simulink model "Simple_RC_Circuit"  (R2024b)
settings: Solver=VariableStepAuto  StartTime=0.0  StopTime=10.0  RelTol=1e-3
values from neighbouring files (symbols this model uses):
  C = 1e-6    (= 1e-06)    [Simple_RC_Circuit_scripit.m]
  R = i    [Simple_RC_Circuit_scripit.m]
settings Model: Creator=Ahmad  LastModifiedBy=Ahmad

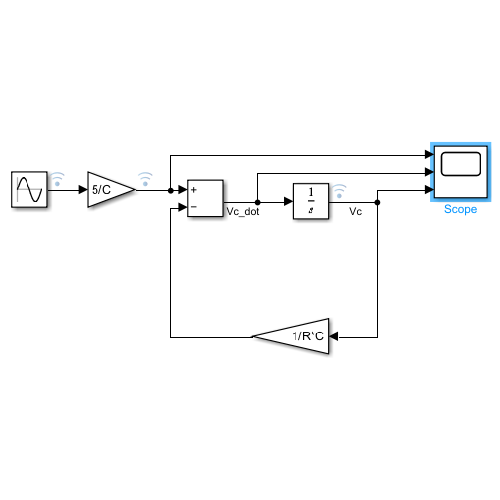
[thumbnail: Simulink's stored preview of the top-level diagram]
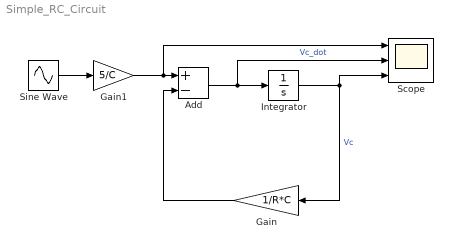
== system Simple_RC_Circuit ==
  Add : Sum  Inputs=+-
  Gain : Gain  Gain=1/R*C
  Gain1 : Gain  Gain=5/C
  Integrator : Integrator
  Scope : Scope  NumInputPorts=3
  Sine Wave : Sin  SampleTime=0
  wires:
  Integrator/1 -> Gain/1, Scope/3  "Vc"
  Gain/1 -> Add/2
  Gain1/1 -> Scope/1, Add/1
  Sine Wave/1 -> Gain1/1
  Add/1 -> Scope/2, Integrator/1  "Vc_dot"
